simulink model "Kalman"  (R2018a)
settings: Solver=VariableStepAuto  StartTime=0.0  StopTime=10.0  RelTol=1e-3
values from neighbouring files (symbols this model uses):
  A = 33    [Lab1.m]    (also in LabB_FInal_version2.mat; Untitled.m)
  C1 = [1 0]    [Lab1.m]    (also in LabB_FInal_version2.mat; Untitled.m)
  C2 = [0 1]    [Lab1.m]    (also in LabB_FInal_version2.mat; Untitled.m)
  K = K'    [Lab1.m]    (also in LabB_FInal_version2.mat = [5.99248777663 0.992989193414]; Untitled.m)
undefined symbols (not defined in the file or in its folder): B
settings Model: Creator=Scott  LastModifiedBy=Scott

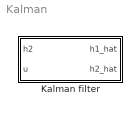
== system Kalman ==
  Kalman filter : Subsystem

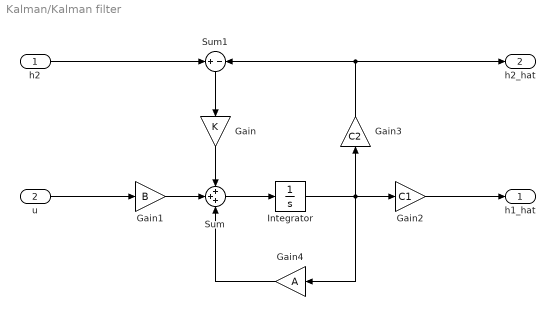
== system Kalman/Kalman filter ==
  h2 : Inport
  u : Inport  Port=2
  Gain : Gain  Gain=K
  Gain1 : Gain  Gain=B
  Gain2 : Gain  Gain=C1
  Gain3 : Gain  Gain=C2
  Gain4 : Gain  Gain=A
  Integrator : Integrator
  Sum : Sum  Inputs=+++
  Sum1 : Sum  Inputs=+|-
  h1_hat : Outport
  h2_hat : Outport  Port=2
  wires:
  u/1 -> Gain1/1
  h2/1 -> Sum1/1
  Integrator/1 -> Gain4/1, Gain3/1, Gain2/1
  Sum/1 -> Integrator/1
  Gain2/1 -> h1_hat/1
  Sum1/1 -> Gain/1
  Gain/1 -> Sum/1
  Gain3/1 -> h2_hat/1, Sum1/2
  Gain4/1 -> Sum/3
  Gain1/1 -> Sum/2
